simulink model "FPC"  (R2024b)
settings: Solver=FixedStepAuto  StartTime=0.0  StopTime=2.4  FixedStep=1e-5  RelTol=1e-3
values from neighbouring files (symbols this model uses):
  dam = 0.707    [data_foc_fpc_zhang.mat]
  DeltaLUT = [-1.14384315458 -1.14384315458 -1.14384315458 -1.14384315458 -1.14384315458 -1.14384315458 -1.14384315458 -1.14384315458 -1.14384315458 -1.14384315458 -1.14384315458 -1.14384315458 ... (19481 elements, 121x161)]    [deltaLUT_plain_zhang.mat]
  gama = 0.9    [data_foc_fpc_zhang.mat]
  imd = [-200 -190 -180 -170 -160 -150 -140 -130 -120 -110 -100 -90 ... (41 elements, 1x41)]    [data_foc_fpc_zhang.mat]
  imq = [-200 -180 -160 -140 -120 -100 -80 -60 -40 -20 0 20 ... (21 elements, 1x21)]    [data_foc_fpc_zhang.mat]
  L_grid = [0.220516868128 0.222482404345 0.224447940562 0.226413476779 0.228379012997 0.230344549214 0.232310085431 0.234275621648 0.236241157866 0.238206694083 0.2401722303 0.242137766517 ... (121 elements, 1x121)]    [deltaLUT_plain_zhang.mat]
  L_loss = 0.0001    [data_foc_fpc_zhang.mat]
  Lmidd = [0.0012418475022 0.00124844926594 0.00125505102968 0.00126370970426 0.00127249900958 0.00128126693334 0.00129343475618 0.00129881592306 0.00130559003385 0.00130625690774 0.00129596814237 0.00127902455887 ... (861 elements, 41x21)]    [data_foc_fpc_zhang.mat]
  Lmidq = [-8.03588800241e-05 -7.81376313538e-05 -7.59163826835e-05 -6.79567507785e-05 -6.10868587727e-05 -5.46820183962e-05 -4.43623922788e-05 -2.78718084301e-05 -1.24477686412e-05 4.13620151953e-06 2.37103656882e-05 4.4707150748e-05 ... (861 elements, 41x21)]    [data_foc_fpc_zhang.mat]
  Lmiqq = [0.000622544120709 0.000618884908772 0.000615225696834 0.000593520125188 0.000579858645255 0.000568946837315 0.000562248369566 0.000560456845994 0.000560437513873 0.000561933244764 0.00056023385138 0.000557379247045 ... (861 elements, 41x21)]    [data_foc_fpc_zhang.mat]
  phase_number = 3    [data_foc_fpc_zhang.mat]
  pp = 4    [data_foc_fpc_zhang.mat]
  Psid = [-0.0498528002107 -0.0378839484092 -0.0259882808465 -0.013034575748 3.54716858652e-05 0.0129865277943 0.0255980427761 0.0386444323153 0.0516254468728 0.0646548336102 0.0777195684651 0.0905974700702 ... (861 elements, 41x21)]    [data_foc_fpc_zhang.mat]
  Psiq = [-0.428836914229 -0.429385909203 -0.42997932915 -0.43118839194 -0.431809140992 -0.432336580454 -0.433057103512 -0.432963079787 -0.433296951787 -0.433632934983 -0.43343561964 -0.433301309559 ... (861 elements, 41x21)]    [data_foc_fpc_zhang.mat]
  Rs = 0.015    [data_foc_fpc_zhang.mat]
  T_grid = [-218.679204233 -215.967777854 -213.256351475 -210.544925095 -207.833498716 -205.122072337 -202.410645958 -199.699219578 -196.987793199 -194.27636682 -191.56494044 -188.853514061 ... (161 elements, 1x161)]    [deltaLUT_plain_zhang.mat]
  T_ref = 162    [data_foc_fpc_zhang.mat]
  Ts = 1e-05    [data_foc_fpc_zhang.mat]
undefined symbols (not defined in the file or in its folder): DiscIntNeverNeededParam, k_fw, lambdaLUT_801, T_break_801, UNC, V_dc
libraries: simulink x8, mcbcontrolslib x4, spsdq0toabcLib x2, simulink_extras x2, eeTransforms x1, spsabctodq0Lib x1, mcbplantlib x1
settings Model: Creator=zhang5  LastModifiedBy=zhang5
settings DataIOCC: ReturnWorkspaceOutputs=off

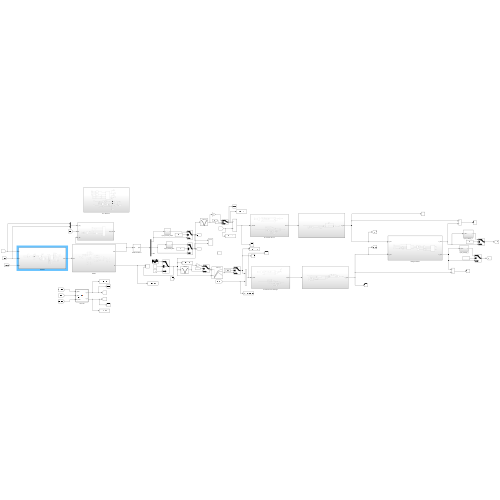
[thumbnail: Simulink's stored preview of the top-level diagram]
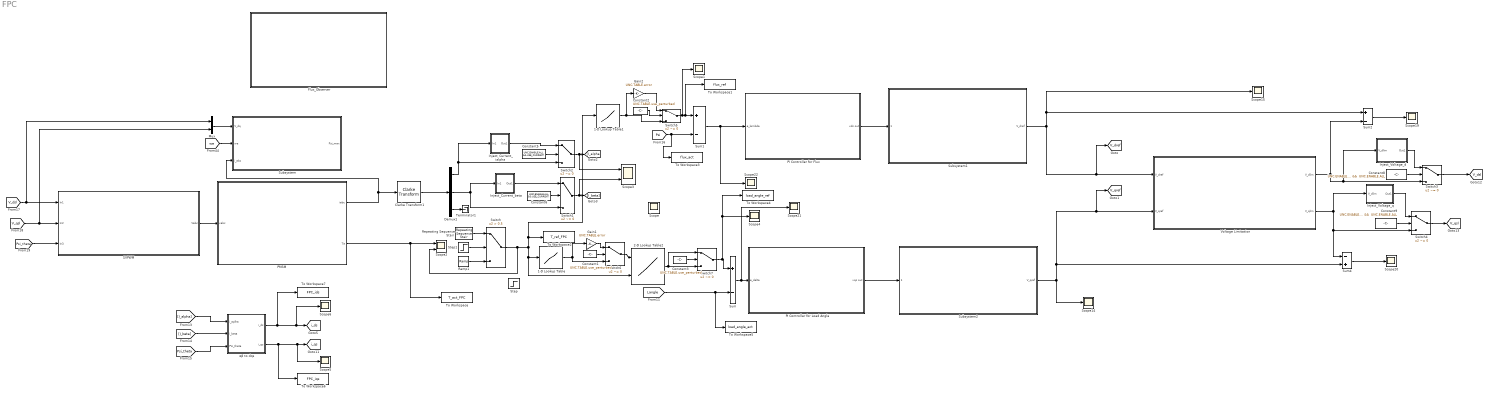
== system FPC ==
  1-D Lookup Table : Lookup_n-D  NumberOfTableDimensions=1  BreakpointsForDimension1=T_break_801  Table=lambdaLUT_801  InternalRulePriority=Speed  RndMeth=Simplest
  1-D Lookup Table1 : Lookup_n-D  NumberOfTableDimensions=1  BreakpointsForDimension1=T_break_801  Table=lambdaLUT_801  InternalRulePriority=Speed  RndMeth=Simplest
  2-D Lookup Table2 : Lookup_n-D  BreakpointsForDimension1=L_grid  BreakpointsForDimension2=T_grid  Table=DeltaLUT  InternalRulePriority=Speed  RndMeth=Simplest
      settings: InputPortMap=u0,u1
  Clarke Transform1 : eeTransforms/Clarke Transform  PowerInvariant=off
      settings: LibrarySourceBlock=|
      | ee_sl_lib/Mathematical
      | Transforms/Clarke Transform
  Constant1 : Constant  Value=UNC.TABLE.use_perturbed
  Constant2 : Constant  Value=UNC.TABLE.use_perturbed
  Constant3 : Constant  Value=UNC.TABLE.use_perturbed
  Constant5 : Constant  Value="UNC.ENABLE.ALL   && USE_CURRENT"
  Constant6 : Constant  Value="UNC.ENABLE.ALL   && USE_CURRENT"
  Constant8 : Constant  Value="UNC.ENABLE.EXEC_DELAY &&  UNC.ENABLE.ALL"
  Constant9 : Constant  Value="UNC.ENABLE.EXEC_DELAY &&  UNC.ENABLE.ALL"
  Demux1 : Demux  Outputs=3
  "Flux_Observer  " : Subsystem
  Gain1 : Gain  Gain=UNC.TABLE.error
  Gain2 : Gain  Gain=UNC.TABLE.error
  Inject_Current_beta : Subsystem
  Inject_Current_ialpha : Subsystem
  Inject_Voltage_d : Subsystem
  Inject_Voltage_q : Subsystem
  Mux : Mux  Inputs=2
  PI Controller for Flux : Subsystem
  "PI Controller for Load Angle " : Subsystem
  PMSM : Subsystem
  Ramp1 : simulink/Sources/Ramp  slope=90  start=0  InitialOutput=0
  Repeating Sequence Stair : simulink/Sources/Repeating Sequence Stair  OutValues=[T_ref -T_ref*0.3 -T_ref*1.8 -T_ref T_ref*1.8 T_ref*0.1].'  tsamp=0.4  OutMin=[]  OutMax=[]  OutDataTypeStr=double  OutputDataTypeScalingMode=double  OutDataType=fixdt(0,8)  ConRadixGroup=Best Precision: Vector-wise  OutScaling=2^-12
  SVPWM : Subsystem
  Scope{,1,4..6,14..15,19..22} (11 alike) : Scope
  Scope2 : Scope  NumInputPorts=2
  Scope3 : Scope  NumInputPorts=2
  Step : Step  Time=0.2  After=162  SampleTime=0
  Step1 : Step  Time=0  SampleTime=0
  Subsystem : Subsystem
  Subsystem1 : Subsystem
  Subsystem2 : Subsystem
  Sum : Sum  Inputs=+-
  Sum1 : Sum  Inputs=+-
  Sum2 : Sum  Inputs=+-
  Sum4 : Sum  Inputs=-+
  Switch : Switch  Criteria=u2 > Threshold  Threshold=0.5  SaturateOnIntegerOverflow=off  InputSameDT=off
  Switch{1..7} (7 alike) : Switch  Criteria=u2 ~= 0  SaturateOnIntegerOverflow=off  InputSameDT=off
  Terminator1 : Terminator
  To Workspace : ToWorkspace  VariableName=T_act_FPC  SaveFormat=Structure With Time  SampleTime=-1
  To Workspace1 : ToWorkspace  VariableName=flux_ref  SaveFormat=Structure With Time  SampleTime=-1
  To Workspace2 : ToWorkspace  VariableName=T_ref_FPC  SaveFormat=Structure With Time  SampleTime=-1
  To Workspace3 : ToWorkspace  VariableName=flux_act  SaveFormat=Structure With Time  SampleTime=-1
  To Workspace4 : ToWorkspace  VariableName=load_angle_ref  SaveFormat=Structure With Time  SampleTime=-1
  To Workspace5 : ToWorkspace  VariableName=load_angle_act  SaveFormat=Structure With Time  SampleTime=-1
  To Workspace6 : ToWorkspace  VariableName=FPC_iqs  SaveFormat=Structure With Time  SampleTime=-1
  To Workspace7 : ToWorkspace  VariableName=FPC_ids  SaveFormat=Structure With Time  SampleTime=-1
  Voltage Limitation : Subsystem
  αβ to dqs : MATLAB Function  TreatAsAtomicUnit=on
  tag scope: V_dref=global, V_dsl=global, V_qref=global, V_qsl=global, i_ds=global, i_qs=global
  wires:
  PMSM/1(iabc) -> Subsystem/3(i_abc), Clarke Transform1/1
  PMSM/2(Te) -> To Workspace/1, Scope2/1
  Clarke Transform1/1 -> Demux1/1
  Demux1/3 -> Terminator1/1
  [Langle] -> To Workspace5/1, Sum/2
  Sum/1 -> Scope21/1, "PI Controller for Load Angle "/1(e_delta)
  [I_alpha] -> αβ to dqs/1(i_aplha)
  [I_beta] -> αβ to dqs/2(i_beta)
  [Psi_theta] -> αβ to dqs/3(Psi_theta)
  αβ to dqs/1(i_ds) -> To Workspace7/1, Scope6/1, [i_ds]
  αβ to dqs/2(i_qs) -> To Workspace6/1, Scope5/1, [i_qs]
  "PI Controller for Load Angle "/1(vqs out) -> Subsystem2/1(" ")
  Subsystem2/1(V_qref) -> [V_qref], Voltage Limitation/2(V_qref), Sum4/2, Scope14/1
  [Psi] -> To Workspace3/1, Sum1/2
  PI Controller for Flux/1(vds out) -> Subsystem1/1(" ")
  Voltage Limitation/1(V_dlim) -> Inject_Voltage_d/1(V_dlim), Switch3/3, Sum2/2
  Sum2/1 -> Scope19/1
  Sum4/1 -> Scope20/1
  Step1/1 -> Switch/2
  Ramp1/1 -> Switch/3
  Repeating Sequence Stair/1 -> Switch/1
  Sum1/1 -> PI Controller for Flux/1(e_lambda), Scope22/1
  Inject_Current_ialpha/1(Out1) -> Switch2/1
  Constant5/1 -> Switch2/2
  Demux1/1 -> Inject_Current_ialpha/1(In1), Switch2/3
  Switch2/1 -> Scope3/1, [I_alpha]
  Demux1/2 -> Switch1/3, Inject_Current_beta/1(In1)
  Constant6/1 -> Switch1/2
  Inject_Current_beta/1(Out1) -> Switch1/1
  Switch1/1 -> Scope3/2, [I_beta]
  Inject_Voltage_d/1(Out1) -> Switch3/1
  Constant8/1 -> Switch3/2
  Switch3/1 -> [V_dsl]
  Constant9/1 -> Switch4/2
  Inject_Voltage_q/1(Out1) -> Switch4/1
  Voltage Limitation/2(V_qlim) -> Switch4/3, Sum4/1, Inject_Voltage_q/1(V_dlim)
  Switch4/1 -> [V_qsl]
  [Psi_theta] -> SVPWM/3(In3)
  [V_dsl] -> Mux/1, SVPWM/1(In1)
  Mux/1 -> Subsystem/1(V_dq)
  [we] -> Subsystem/2(we)
  [V_qsl] -> Mux/2, SVPWM/2(In2)
  SVPWM/1(Vabc) -> PMSM/1(vabc)
  Subsystem1/1(V_dref) -> Sum2/1, Scope15/1, [V_dref], Voltage Limitation/1(V_dref)
  Switch/1 -> Scope2/2, 1-D Lookup Table1/1, To Workspace2/1, 2-D Lookup Table2/2, 1-D Lookup Table/1
  Gain2/1 -> Switch5/1
  Constant2/1 -> Switch5/2
  1-D Lookup Table1/1 -> Gain2/1, Switch5/3
  Switch5/1 -> Scope1/1, To Workspace1/1, Sum1/1
  Switch6/1 -> 2-D Lookup Table2/1
  Constant1/1 -> Switch6/2
  1-D Lookup Table/1 -> Gain1/1, Switch6/3
  Gain1/1 -> Switch6/1
  Switch7/1 -> Scope4/1, To Workspace4/1, Sum/1
  2-D Lookup Table2/1 -> Switch7/1, Switch7/3
  Constant3/1 -> Switch7/2

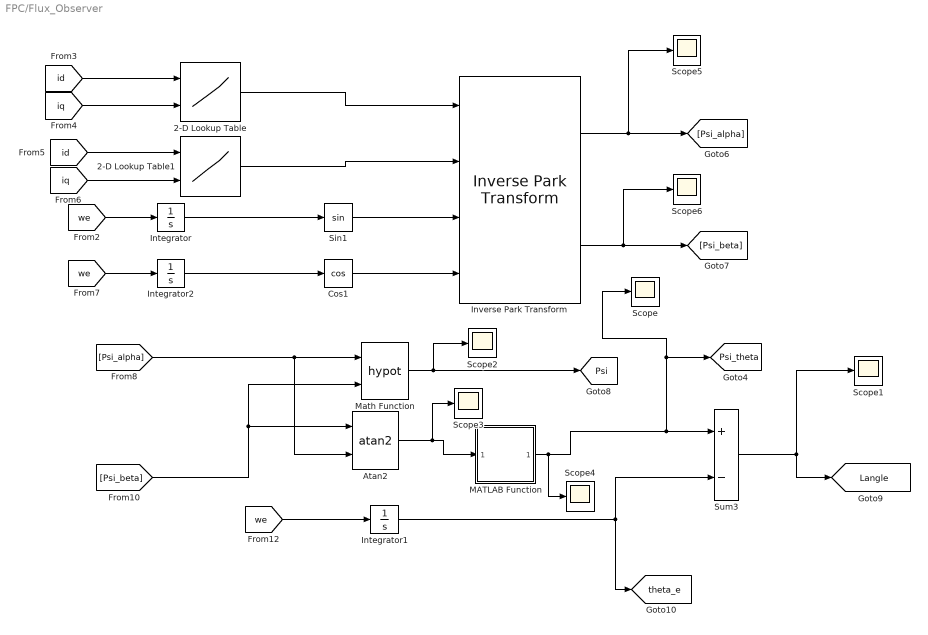
== system FPC/Flux_Observer   ==
  2-D Lookup Table : Lookup_n-D  BreakpointsForDimension1=imd  BreakpointsForDimension2=imq  Table=Psid  InternalRulePriority=Speed  RndMeth=Simplest
      settings: InputPortMap=u0,u1
  2-D Lookup Table1 : Lookup_n-D  BreakpointsForDimension1=imd  BreakpointsForDimension2=imq  Table=Psiq  InternalRulePriority=Speed  RndMeth=Simplest
      settings: InputPortMap=u0,u1
  Atan2 : Trigonometry  Operator=atan2
  Cos1 : Trigonometry  Operator=cos
  Integrator : Integrator
  Integrator1 : Integrator
  Integrator2 : Integrator
  Inverse Park Transform : mcbcontrolslib/Inverse Park Transform  PhaseInput=Two inputs  AxisAlignment=D-axis  ThetaInput=Sine and Cosine electrical position  AngleInput=Per-unit  N_points=1024
      settings: LibrarySourceBlock=mcblib/Controls/Math Transforms/Inverse Park Transform
  MATLAB Function : MATLAB Function  TreatAsAtomicUnit=on
  Math Function : Math  Operator=hypot
  Scope{,1..6} (7 alike) : Scope
  Sin1 : Trigonometry
  Sum3 : Sum  Inputs=+-
  tag scope: Langle=global, Psi=global, Psi_theta=global, theta_e=global
  wires:
  [id] -> 2-D Lookup Table1/1
  MATLAB Function/1(theta_u) -> Scope4/1, [Psi_theta], Scope/1, Sum3/1
  Inverse Park Transform/1 -> Scope5/1, [Psi_alpha]
  [Psi_alpha] -> Atan2/2, Math Function/1
  Integrator2/1 -> Cos1/1
  2-D Lookup Table1/1 -> Inverse Park Transform/2
  [Psi_beta] -> Atan2/1, Math Function/2
  Sin1/1 -> Inverse Park Transform/3
  Integrator/1 -> Sin1/1
  Cos1/1 -> Inverse Park Transform/4
  Integrator1/1 -> [theta_e], Sum3/2
  [we] -> Integrator1/1
  Math Function/1 -> Scope2/1, [Psi]
  Inverse Park Transform/2 -> Scope6/1, [Psi_beta]
  Sum3/1 -> [Langle], Scope1/1
  [iq] -> 2-D Lookup Table/2
  2-D Lookup Table/1 -> Inverse Park Transform/1
  [iq] -> 2-D Lookup Table1/2
  [we] -> Integrator/1
  [we] -> Integrator2/1
  [id] -> 2-D Lookup Table/1
  Atan2/1 -> Scope3/1, MATLAB Function/1(theta_w)

== system FPC/Inject_Current_beta ==
  In1 : Inport
  Band-Limited White Noise : simulink/Sources/Band-Limited White Noise  Cov=UNC.CURR.noise_psd  Ts=1e-5  seed=[23341]
  Bias : Bias  Bias=UNC.CURR.bias_alpha  SaturateOnIntegerOverflow=off
  Quantizer : Quantizer  QuantizationInterval=UNC.CURR.quant
  Sum4 : Sum
  Out1 : Outport
  wires:
  Sum4/1 -> Quantizer/1
  Quantizer/1 -> Out1/1
  In1/1 -> Bias/1
  Bias/1 -> Sum4/1
  Band-Limited White Noise/1 -> Sum4/2

== system FPC/Inject_Current_ialpha ==
  In1 : Inport
  Band-Limited White Noise : simulink/Sources/Band-Limited White Noise  Cov=UNC.CURR.noise_psd  Ts=1e-5  seed=[23341]
  Bias : Bias  Bias=UNC.CURR.bias_alpha  SaturateOnIntegerOverflow=off
  Quantizer : Quantizer  QuantizationInterval=UNC.CURR.quant
  Sum4 : Sum
  Out1 : Outport
  wires:
  Band-Limited White Noise/1 -> Sum4/2
  Bias/1 -> Sum4/1
  In1/1 -> Bias/1
  Quantizer/1 -> Out1/1
  Sum4/1 -> Quantizer/1

== system FPC/Inject_Voltage_d ==
  V_dlim : Inport
  Transport Delay : TransportDelay  DelayTime=UNC.DELAY.ctrl
  Out1 : Outport
  wires:
  Transport Delay/1 -> Out1/1
  V_dlim/1 -> Transport Delay/1

== system FPC/Inject_Voltage_q ==
  V_dlim : Inport
  Transport Delay : TransportDelay  DelayTime=UNC.DELAY.ctrl
  Out1 : Outport
  wires:
  V_dlim/1 -> Transport Delay/1
  Transport Delay/1 -> Out1/1

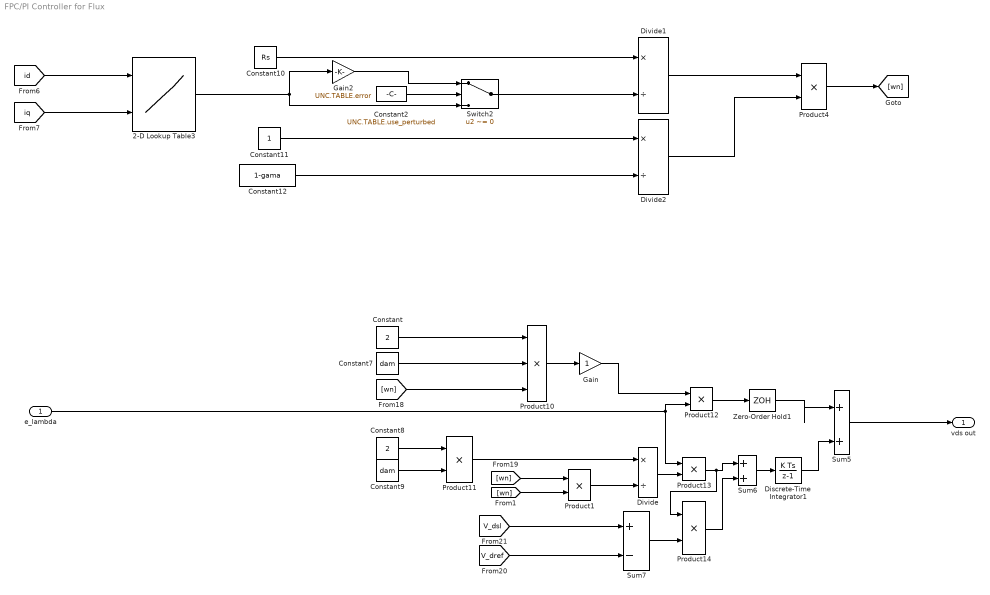
== system FPC/PI Controller for Flux ==
  e_lambda : Inport
  2-D Lookup Table3 : Lookup_n-D  BreakpointsForDimension1=imd  BreakpointsForDimension2=imq  Table=Lmidd  InternalRulePriority=Speed  RndMeth=Simplest
      settings: InputPortMap=u0,u1
  Constant : Constant  Value=2
  Constant10 : Constant  Value=Rs
  Constant11 : Constant
  Constant12 : Constant  Value=1-gama
  Constant2 : Constant  Value=UNC.TABLE.use_perturbed
  Constant7 : Constant  Value=dam
  Constant8 : Constant  Value=2
  Constant9 : Constant  Value=dam
  Discrete-Time Integrator1 : DiscreteIntegrator  SampleTime=Ts  ICPrevOutput=DiscIntNeverNeededParam  ICPrevScaledInput=DiscIntNeverNeededParam
  Divide : Product  Inputs=*/
  Divide1 : Product  Inputs=*/
  Divide2 : Product  Inputs=*/
  Gain : Gain
  Gain2 : Gain  Gain=UNC.TABLE.error
  Product{1,4,11..14} (6 alike) : Product
  Product10 : Product  Inputs=3
  Sum5 : Sum  Inputs=|++
  Sum6 : Sum
  Sum7 : Sum  Inputs=+-
  Switch2 : Switch  Criteria=u2 ~= 0  SaturateOnIntegerOverflow=off  InputSameDT=off
  Zero-Order Hold1 : ZeroOrderHold  SampleTime=Ts
  vds out : Outport
  wires:
  Divide/1 -> Product13/2
  Product12/1 -> Zero-Order Hold1/1
  e_lambda/1 -> Product12/2, Product13/1
  Product10/1 -> Gain/1
  Product11/1 -> Divide/1
  Constant9/1 -> Product11/2
  Constant8/1 -> Product11/1
  [wn] -> Product10/3
  Constant7/1 -> Product10/2
  Constant/1 -> Product10/1
  Sum5/1 -> vds out/1
  Discrete-Time Integrator1/1 -> Sum5/2
  Zero-Order Hold1/1 -> Sum5/1
  Constant12/1 -> Divide2/2
  Divide2/1 -> Product4/2
  Constant11/1 -> Divide2/1
  Divide1/1 -> Product4/1
  [id] -> 2-D Lookup Table3/1
  [iq] -> 2-D Lookup Table3/2
  Constant10/1 -> Divide1/1
  Sum6/1 -> Discrete-Time Integrator1/1
  Product13/1 -> Product14/1, Sum6/1
  Sum7/1 -> Product14/2
  [V_dsl] -> Sum7/1
  [V_dref] -> Sum7/2
  Product14/1 -> Sum6/2
  Product4/1 -> [wn]
  Gain/1 -> Product12/1
  Constant2/1 -> Switch2/2
  Gain2/1 -> Switch2/1
  2-D Lookup Table3/1 -> Switch2/3, Gain2/1
  Switch2/1 -> Divide1/2
  [wn] -> Product1/1
  Product1/1 -> Divide/2
  [wn] -> Product1/2

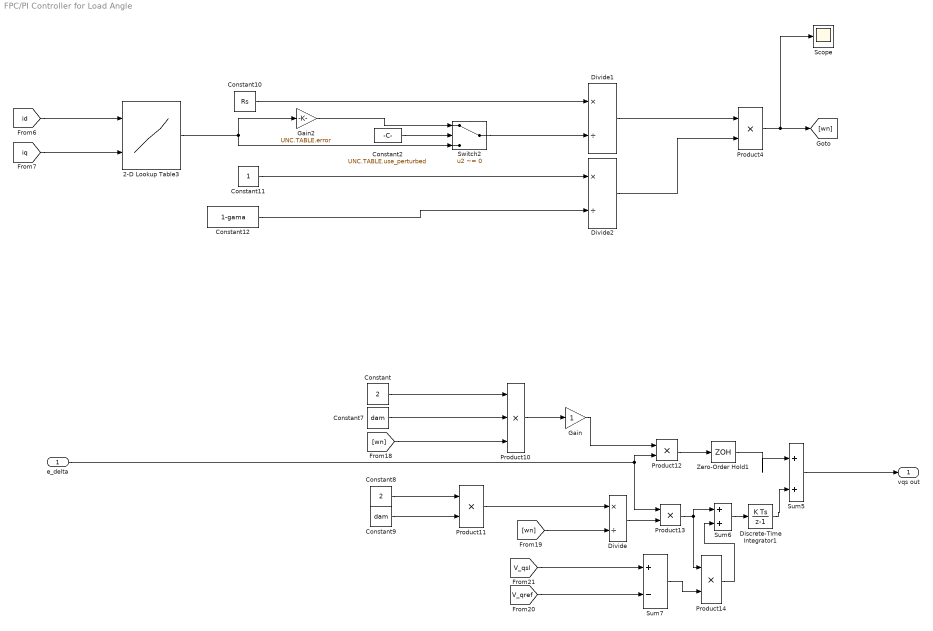
== system FPC/PI Controller for Load Angle  ==
  e_delta : Inport
  2-D Lookup Table3 : Lookup_n-D  BreakpointsForDimension1=imd  BreakpointsForDimension2=imq  Table=Lmiqq  InternalRulePriority=Speed  RndMeth=Simplest
      settings: InputPortMap=u0,u1
  Constant : Constant  Value=2
  Constant10 : Constant  Value=Rs
  Constant11 : Constant
  Constant12 : Constant  Value=1-gama
  Constant2 : Constant  Value=UNC.TABLE.use_perturbed
  Constant7 : Constant  Value=dam
  Constant8 : Constant  Value=2
  Constant9 : Constant  Value=dam
  Discrete-Time Integrator1 : DiscreteIntegrator  SampleTime=Ts  ICPrevOutput=DiscIntNeverNeededParam  ICPrevScaledInput=DiscIntNeverNeededParam
  Divide : Product  Inputs=*/
  Divide1 : Product  Inputs=*/
  Divide2 : Product  Inputs=*/
  Gain : Gain
  Gain2 : Gain  Gain=UNC.TABLE.error
  Product10 : Product  Inputs=3
  Product{4,11..14} (5 alike) : Product
  Scope : Scope
  Sum5 : Sum  Inputs=|++
  Sum6 : Sum
  Sum7 : Sum  Inputs=+-
  Switch2 : Switch  Criteria=u2 ~= 0  SaturateOnIntegerOverflow=off  InputSameDT=off
  Zero-Order Hold1 : ZeroOrderHold  SampleTime=Ts
  vqs out : Outport
  wires:
  Constant10/1 -> Divide1/1
  [iq] -> 2-D Lookup Table3/2
  [id] -> 2-D Lookup Table3/1
  Divide1/1 -> Product4/1
  Product4/1 -> Scope/1, [wn]
  Constant11/1 -> Divide2/1
  Divide2/1 -> Product4/2
  Constant12/1 -> Divide2/2
  Zero-Order Hold1/1 -> Sum5/1
  Discrete-Time Integrator1/1 -> Sum5/2
  Sum5/1 -> vqs out/1
  Constant/1 -> Product10/1
  Constant7/1 -> Product10/2
  [wn] -> Product10/3
  Constant8/1 -> Product11/1
  Constant9/1 -> Product11/2
  Product11/1 -> Divide/1
  [wn] -> Divide/2
  Product10/1 -> Gain/1
  e_delta/1 -> Product13/1, Product12/2
  Product12/1 -> Zero-Order Hold1/1
  Divide/1 -> Product13/2
  Product13/1 -> Product14/1, Sum6/1
  [V_qref] -> Sum7/2
  [V_qsl] -> Sum7/1
  Sum7/1 -> Product14/2
  Sum6/1 -> Discrete-Time Integrator1/1
  Product14/1 -> Sum6/2
  Gain/1 -> Product12/1
  Constant2/1 -> Switch2/2
  Gain2/1 -> Switch2/1
  2-D Lookup Table3/1 -> Switch2/3, Gain2/1
  Switch2/1 -> Divide1/2

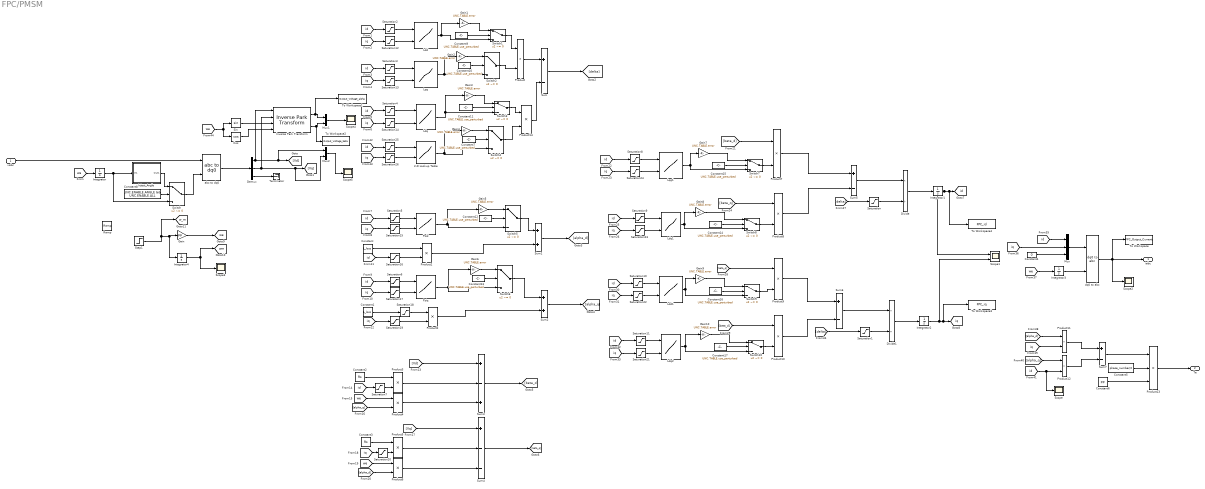
== system FPC/PMSM ==
  vabc : Inport
  2-D Lookup Table : Lookup_n-D  BreakpointsForDimension1=imd  BreakpointsForDimension2=imq  Table=Lmidq  ExtrapMethod=Clip  UseLastTableValue=on  InternalRulePriority=Speed  RndMeth=Simplest
      settings: InputPortMap=u0,u1
  Constant : Constant  Value=L_loss
  Constant1 : Constant  Value=L_loss
  Constant{7,9..17} (10 alike) : Constant  Value=UNC.TABLE.use_perturbed
  Constant2 : Constant  Value=Rs
  Constant3 : Constant  Value=Rs
  Constant4 : Constant  Value=0
  Constant5 : Constant  Value=phase_number/2
  Constant6 : Constant  Value=pp
  Constant8 : Constant  Value=UNC.ENABLE.ANGLE && UNC.ENABLE.ALL
  Cos : Trigonometry  Operator=cos
  Demux : Demux  Outputs=3
  Divide : Product  Inputs=*/
  Divide1 : Product  Inputs=*/
  Gain : Gain  Gain=pp
  Gain{1..10} (10 alike) : Gain  Gain=UNC.TABLE.error
  Inject_Angle : Subsystem
  Integrator : Integrator  UpperSaturationLimit=pi  LowerSaturationLimit=-pi
  Integrator1 : Integrator
  Integrator2 : Integrator
  Integrator3 : Integrator  UpperSaturationLimit=pi  LowerSaturationLimit=-pi
  Integrator4 : Integrator
  Inverse Park Transform : mcbcontrolslib/Inverse Park Transform  PhaseInput=Two inputs  AxisAlignment=D-axis  ThetaInput=Sine and Cosine electrical position  AngleInput=Per-unit  N_points=1024
      settings: LibrarySourceBlock=mcbhdllib/Controls/Math Transforms/Inverse Park Transform
  Ldd : Lookup_n-D  BreakpointsForDimension1=imd  BreakpointsForDimension2=imq  Table=Lmidd  ExtrapMethod=Clip  UseLastTableValue=on  InternalRulePriority=Speed  RndMeth=Simplest
      settings: InputPortMap=u0,u1
  Ldd1 : Lookup_n-D  BreakpointsForDimension1=imd  BreakpointsForDimension2=imq  Table=Lmidd  ExtrapMethod=Clip  UseLastTableValue=on  InternalRulePriority=Speed  RndMeth=Simplest
      settings: InputPortMap=u0,u1
  Ldq : Lookup_n-D  BreakpointsForDimension1=imd  BreakpointsForDimension2=imq  Table=Lmidq  ExtrapMethod=Clip  UseLastTableValue=on  InternalRulePriority=Speed  RndMeth=Simplest
      settings: InputPortMap=u0,u1
  Ldq1 : Lookup_n-D  BreakpointsForDimension1=imd  BreakpointsForDimension2=imq  Table=Lmidq  ExtrapMethod=Clip  UseLastTableValue=on  InternalRulePriority=Speed  RndMeth=Simplest
      settings: InputPortMap=u0,u1
  Ldq2 : Lookup_n-D  BreakpointsForDimension1=imd  BreakpointsForDimension2=imq  Table=Lmidq  ExtrapMethod=Clip  UseLastTableValue=on  InternalRulePriority=Speed  RndMeth=Simplest
      settings: InputPortMap=u0,u1
  Lqq : Lookup_n-D  BreakpointsForDimension1=imd  BreakpointsForDimension2=imq  Table=Lmiqq  ExtrapMethod=Clip  UseLastTableValue=on  InternalRulePriority=Speed  RndMeth=Simplest
      settings: InputPortMap=u0,u1
  Lqq1 : Lookup_n-D  BreakpointsForDimension1=imd  BreakpointsForDimension2=imq  Table=Lmiqq  ExtrapMethod=Clip  UseLastTableValue=on  InternalRulePriority=Speed  RndMeth=Simplest
      settings: InputPortMap=u0,u1
  Mux : Mux  Inputs=3
  Mux1 : Mux  Inputs=2
  Mux2 : Mux  Inputs=2
  Product{,1..12,14} (14 alike) : Product
  Product13 : Product  Inputs=3
  Psid : Lookup_n-D  BreakpointsForDimension1=imd  BreakpointsForDimension2=imq  Table=Psid  ExtrapMethod=Clip  UseLastTableValue=on  InternalRulePriority=Speed  RndMeth=Simplest
      settings: InputPortMap=u0,u1
  Psiq : Lookup_n-D  BreakpointsForDimension1=imd  BreakpointsForDimension2=imq  Table=Psiq  ExtrapMethod=Clip  UseLastTableValue=on  InternalRulePriority=Speed  RndMeth=Simplest
      settings: InputPortMap=u0,u1
  Ramp : simulink/Sources/Ramp  slope=8.9757  start=0  InitialOutput=0
  Saturation : Saturate  UpperLimit=10000000000000000000000  LowerLimit=1e-6
  Saturation1 : Saturate  UpperLimit=10000000000000000000000  LowerLimit=1e-6
  Saturation{2..11,13..26} (24 alike) : Saturate  UpperLimit=200  LowerLimit=-200
  Saturation12 : Saturate
  Scope{,2..5} (5 alike) : Scope
  Scope1 : Scope  NumInputPorts=2
  Sin : Trigonometry
  Step1 : Step  Time=5  Before=10.4720 * 2  After=10.4720*1.2  SampleTime=0
  Sum{,5..7} (4 alike) : Sum  Inputs=+-
  Sum1 : Sum
  Sum2 : Sum
  Sum3 : Sum  Inputs=+-+
  Sum4 : Sum  Inputs=+--
  Switch{,1..10} (11 alike) : Switch  Criteria=u2 ~= 0  SaturateOnIntegerOverflow=off  InputSameDT=off
  Terminator : Terminator
  To Workspace : ToWorkspace  VariableName=FPC_Output_Current  SaveFormat=Timeseries  SampleTime=-1
  To Workspace1 : ToWorkspace  VariableName=Output_Voltage_alpha  SaveFormat=Structure With Time  SampleTime=-1
  To Workspace2 : ToWorkspace  VariableName=Output_Voltage_beta  SaveFormat=Structure With Time  SampleTime=-1
  To Workspace3 : ToWorkspace  VariableName=FPC_iq  SaveFormat=Structure With Time  SampleTime=-1
  To Workspace4 : ToWorkspace  VariableName=FPC_id  SaveFormat=Structure With Time  SampleTime=-1
  abc to dq0 : spsabctodq0Lib/abc to dq0  Alignment=Aligned with phase A axis
  dq0 to abc : spsdq0toabcLib/dq0 to abc  Alignment=Aligned with phase A axis
  iabc : Outport
  Te : Outport  Port=2
  tag scope: id=global, iq=global, w_m=global, we=global, wm=global
  wires:
  Product1/1 -> Sum1/2
  abc to dq0/1 -> Demux/1
  Demux/2 -> Inverse Park Transform/2, Mux2/2, [Vq]
  Demux/1 -> Inverse Park Transform/1, Mux2/1, [Vd]
  Product2/1 -> Sum2/2
  Saturation26/1 -> 2-D Lookup Table/2
  Saturation25/1 -> 2-D Lookup Table/1
  [iq] -> Saturation26/1
  [id] -> Saturation25/1
  Saturation24/1 -> Lqq1/2
  Saturation23/1 -> Ldq1/2
  Saturation22/1 -> Ldd1/2
  Saturation21/1 -> Ldq2/2
  Saturation20/1 -> Product5/2
  Saturation19/1 -> Product2/2
  Saturation18/1 -> Product2/1
  Saturation17/1 -> Psiq/2
  Saturation16/1 -> Product1/2
  Saturation15/1 -> Psid/2
  Saturation14/1 -> Ldq/2
  Saturation13/1 -> Lqq/2
  Saturation12/1 -> Ldd/2
  Saturation11/1 -> Ldq2/1
  Saturation10/1 -> Ldd1/1
  Saturation9/1 -> Ldq1/1
  Saturation8/1 -> Lqq1/1
  Saturation7/1 -> Product3/2
  Saturation6/1 -> Psiq/1
  Saturation5/1 -> Psid/1
  Saturation4/1 -> Ldq/1
  Saturation3/1 -> Lqq/1
  Saturation2/1 -> Ldd/1
  Saturation1/1 -> Divide1/2
  Saturation/1 -> Divide/2
  Product13/1 -> Te/1
  Constant6/1 -> Product13/3
  Constant5/1 -> Product13/2
  Sum7/1 -> Product13/1
  Product12/1 -> Sum7/2
  [id] -> Product12/2, Scope/1
  [alpha_q] -> Product12/1
  Product11/1 -> Sum7/1
  [iq] -> Product11/2
  [alpha_d] -> Product11/1
  [beta_q] -> Product9/1
  [iq] -> Saturation22/1
  Sum/1 -> [delta]
  Constant/1 -> Product1/1
  Integrator1/1 -> Scope1/1, To Workspace4/1, [id]
  [delta] -> Saturation1/1
  [Vd] -> Sum3/1
  [id] -> Saturation5/1
  [id] -> Saturation11/1
  Sum1/1 -> [alpha_d]
  Sum4/1 -> [beta_q]
  [alpha_q] -> Product4/2
  Sum3/1 -> [beta_d]
  [we] -> Product6/1
  Sum6/1 -> Divide1/1
  Product/1 -> Sum/1
  [iq] -> Saturation23/1
  [we] -> Product4/1
  [id] -> Mux/1
  Product10/1 -> Sum6/2
  Constant1/1 -> Saturation18/1
  Product5/1 -> Sum4/2
  Product9/1 -> Sum6/1
  Divide/1 -> Integrator1/1
  [iq] -> Mux/2
  [id] -> Saturation8/1
  [beta_d] -> Product7/1
  Integrator2/1 -> To Workspace3/1, [iq], Scope1/2
  Integrator3/1 -> dq0 to abc/2
  [beta_q] -> Product8/1
  Gain/1 -> [we]
  Product3/1 -> Sum3/2
  Product8/1 -> Sum5/2
  Sum5/1 -> Divide/1
  [id] -> Saturation7/1
  [delta] -> Saturation/1
  [we] -> Integrator3/1
  [iq] -> Saturation20/1
  [id] -> Saturation4/1
  Product14/1 -> Sum/2
  Sum2/1 -> [alpha_q]
  Product7/1 -> Sum5/1
  [iq] -> Saturation24/1
  [id] -> Saturation3/1
  [iq] -> Saturation13/1
  Product6/1 -> Sum4/3
  [id] -> Saturation9/1
  Mux/1 -> dq0 to abc/1
  [iq] -> Saturation14/1
  [alpha_d] -> Product6/2
  Divide1/1 -> Integrator2/1
  [Vq] -> Sum4/1
  [id] -> Saturation6/1
  Constant4/1 -> Mux/3
  dq0 to abc/1 -> To Workspace/1, iabc/1, Scope2/1
  Demux/3 -> Terminator/1
  [id] -> Saturation10/1
  [we] -> Integrator/1
  [beta_d] -> Product10/1
  [id] -> Saturation2/1
  Constant3/1 -> Product5/1
  [id] -> Saturation16/1
  [iq] -> Saturation15/1
  [iq] -> Saturation19/1
  Product4/1 -> Sum3/3
  Constant2/1 -> Product3/1
  [iq] -> Saturation21/1
  [iq] -> Saturation12/1
  [iq] -> Saturation17/1
  vabc/1 -> abc to dq0/1
  Step1/1 -> Gain/1, Integrator4/1, [w_m]
  Constant8/1 -> Switch/2
  Inject_Angle/1(Out1) -> Switch/1
  Integrator/1 -> Switch/3, Inject_Angle/1(In1)
  Integrator4/1 -> Scope3/1, [wm]
  Switch/1 -> abc to dq0/2
  Constant10/1 -> Switch2/2
  Switch2/1 -> Product/2
  Gain2/1 -> Switch2/1
  Gain1/1 -> Switch1/1
  Constant9/1 -> Switch1/2
  Ldd/1 -> Gain1/1, Switch1/3
  Lqq/1 -> Switch2/3, Gain2/1
  Switch1/1 -> Product/1
  2-D Lookup Table/1 -> Gain4/1, Switch4/3
  Ldq/1 -> Switch3/3, Gain3/1
  Constant11/1 -> Switch3/2
  Gain3/1 -> Switch3/1
  Gain4/1 -> Switch4/1
  Switch4/1 -> Product14/2
  Constant7/1 -> Switch4/2
  Switch3/1 -> Product14/1
  Constant12/1 -> Switch5/2
  Gain5/1 -> Switch5/1
  Psid/1 -> Gain5/1, Switch5/3
  Switch5/1 -> Sum1/1
  Switch6/1 -> Sum2/1
  Psiq/1 -> Switch6/3, Gain6/1
  Gain6/1 -> Switch6/1
  Constant13/1 -> Switch6/2
  Constant15/1 -> Switch7/2
  Gain7/1 -> Switch7/1
  Lqq1/1 -> Switch7/3, Gain7/1
  Switch7/1 -> Product7/2
  Ldq1/1 -> Gain8/1, Switch8/3
  Gain8/1 -> Switch8/1
  Constant14/1 -> Switch8/2
  Switch8/1 -> Product8/2
  Constant16/1 -> Switch9/2
  Gain9/1 -> Switch9/1
  Ldd1/1 -> Switch9/3, Gain9/1
  Switch9/1 -> Product9/2
  Ldq2/1 -> Switch10/3, Gain10/1
  Gain10/1 -> Switch10/1
  Constant17/1 -> Switch10/2
  Switch10/1 -> Product10/2
  Sin/1 -> Inverse Park Transform/3
  [we] -> Cos/1, Sin/1
  Cos/1 -> Inverse Park Transform/4
  Inverse Park Transform/1 -> To Workspace1/1, Mux1/1
  Inverse Park Transform/2 -> To Workspace2/1, Mux1/2
  Mux1/1 -> Scope4/1
  Mux2/1 -> Scope5/1

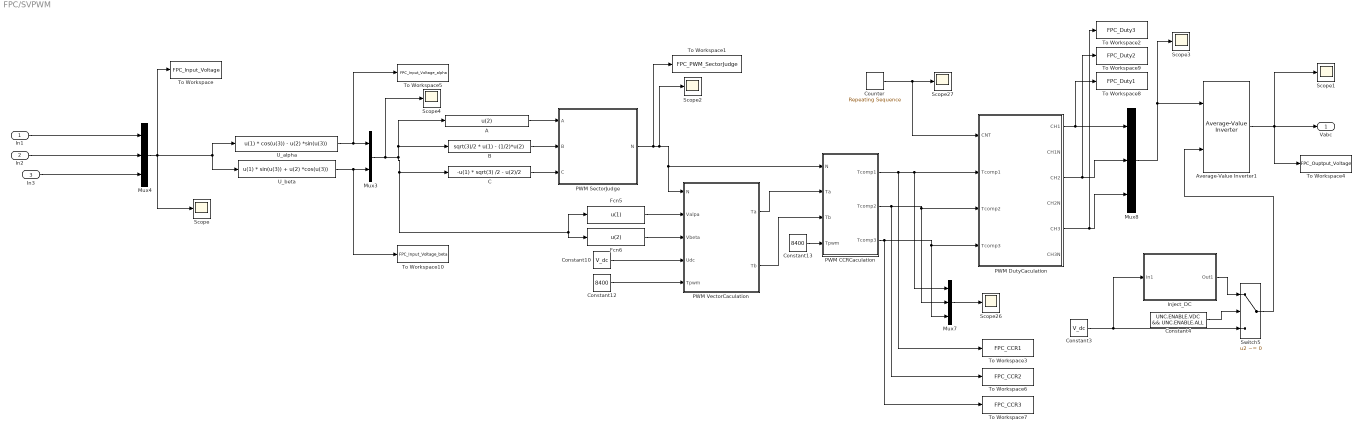
== system FPC/SVPWM ==
  In1 : Inport
  In2 : Inport  Port=2
  In3 : Inport  Port=3
  A : Fcn  Expr=u(2)
  Average-Value Inverter1 : mcbplantlib/Average-Value Inverter
      settings: LibrarySourceBlock=mcblib/Electrical Systems/Inverters/Average-Value Inverter
  B : Fcn  Expr=sqrt(3)/2 * u(1) - (1/2)*u(2)
  C : Fcn  Expr=-u(1) * sqrt(3) /2 - u(2)/2
  Constant10 : Constant  Value=V_dc
  Constant12 : Constant  Value=8400
  Constant13 : Constant  Value=8400
  Constant3 : Constant  Value=V_dc
  Constant4 : Constant  Value=UNC.ENABLE.VDC && UNC.ENABLE.ALL
  Counter : simulink/Sources/Repeating Sequence  rep_seq_t=[0 0.00025 0.0005]  rep_seq_y=[0 4200 0]
  Fcn5 : Fcn  Expr=u(1)
  Fcn6 : Fcn  Expr=u(2)
  Inject_DC : Subsystem
  Mux3 : Mux  Inputs=2
  Mux4 : Mux  Inputs=3
  Mux7 : Mux  Inputs=3
  Mux8 : Mux  Inputs=3
  PWM CCRCaculation : MATLAB Function  TreatAsAtomicUnit=on
  PWM DutyCaculation : MATLAB Function  TreatAsAtomicUnit=on
  PWM SectorJudge : MATLAB Function  TreatAsAtomicUnit=on
  PWM VectorCaculation : MATLAB Function  TreatAsAtomicUnit=on
  Scope{,1..4,26..27} (7 alike) : Scope
  Switch5 : Switch  Criteria=u2 ~= 0  SaturateOnIntegerOverflow=off  InputSameDT=off
  To Workspace : ToWorkspace  VariableName=FPC_Input_Voltage  SaveFormat=Structure With Time  SampleTime=-1
  To Workspace1 : ToWorkspace  VariableName=FPC_PWM_SectorJudge  SaveFormat=Structure With Time  SampleTime=-1
  To Workspace10 : ToWorkspace  VariableName=FPC_Input_Voltage_beta  SaveFormat=Structure With Time  SampleTime=-1
  To Workspace2 : ToWorkspace  VariableName=FPC_Duty3  SaveFormat=Structure With Time  SampleTime=-1
  To Workspace3 : ToWorkspace  VariableName=FPC_CCR1  SaveFormat=Structure With Time  SampleTime=-1
  To Workspace4 : ToWorkspace  VariableName=FPC_Ouptput_Voltage  SaveFormat=Structure With Time  SampleTime=-1
  To Workspace5 : ToWorkspace  VariableName=FPC_Input_Voltage_alpha  SaveFormat=Structure With Time  SampleTime=-1
  To Workspace6 : ToWorkspace  VariableName=FPC_CCR2  SaveFormat=Structure With Time  SampleTime=-1
  To Workspace7 : ToWorkspace  VariableName=FPC_CCR3  SaveFormat=Structure With Time  SampleTime=-1
  To Workspace8 : ToWorkspace  VariableName=FPC_Duty1  SaveFormat=Structure With Time  SampleTime=-1
  To Workspace9 : ToWorkspace  VariableName=FPC_Duty2  SaveFormat=Structure With Time  SampleTime=-1
  U_alpha : Fcn  Expr=u(1) * cos(u(3)) - u(2) *sin(u(3))
  U_beta : Fcn  Expr=u(1) * sin(u(3)) + u(2) *cos(u(3))
  Vabc : Outport
  wires:
  PWM CCRCaculation/1(Tcomp1) -> To Workspace3/1, Mux7/1, PWM DutyCaculation/2(Tcomp1)
  PWM DutyCaculation/5(CH3) -> To Workspace2/1, Mux8/3
  Mux3/1 -> Scope4/1, Fcn6/1, Fcn5/1, C/1, A/1, B/1
  B/1 -> PWM SectorJudge/2(B)
  PWM SectorJudge/1(N) -> To Workspace1/1, Scope2/1, PWM VectorCaculation/1(N), PWM CCRCaculation/1(N)
  Mux4/1 -> Scope/1, To Workspace/1, U_beta/1, U_alpha/1
  Constant3/1 -> Switch5/3, Inject_DC/1(In1)
  Counter/1 -> Scope27/1, PWM DutyCaculation/1(CNT)
  Constant4/1 -> Switch5/2
  Inject_DC/1(Out1) -> Switch5/1
  PWM DutyCaculation/1(CH1) -> To Workspace8/1, Mux8/1
  Constant10/1 -> PWM VectorCaculation/4(Udc)
  PWM DutyCaculation/3(CH2) -> To Workspace9/1, Mux8/2
  U_beta/1 -> To Workspace10/1, Mux3/2
  Constant13/1 -> PWM CCRCaculation/4(Tpwm)
  Fcn6/1 -> PWM VectorCaculation/3(Vbeta)
  C/1 -> PWM SectorJudge/3(C)
  A/1 -> PWM SectorJudge/1(A)
  PWM CCRCaculation/2(Tcomp2) -> To Workspace6/1, Mux7/2, PWM DutyCaculation/3(Tcomp2)
  Mux7/1 -> Scope26/1
  U_alpha/1 -> To Workspace5/1, Mux3/1
  Constant12/1 -> PWM VectorCaculation/5(Tpwm)
  PWM VectorCaculation/2(Tb) -> PWM CCRCaculation/3(Tb)
  PWM CCRCaculation/3(Tcomp3) -> To Workspace7/1, Mux7/3, PWM DutyCaculation/4(Tcomp3)
  In1/1 -> Mux4/1
  Switch5/1 -> Average-Value Inverter1/2
  Fcn5/1 -> PWM VectorCaculation/2(Valpa)
  Mux8/1 -> Scope3/1, Average-Value Inverter1/1
  PWM VectorCaculation/1(Ta) -> PWM CCRCaculation/2(Ta)
  In3/1 -> Mux4/3
  In2/1 -> Mux4/2
  Average-Value Inverter1/1 -> Scope1/1, Vabc/1, To Workspace4/1

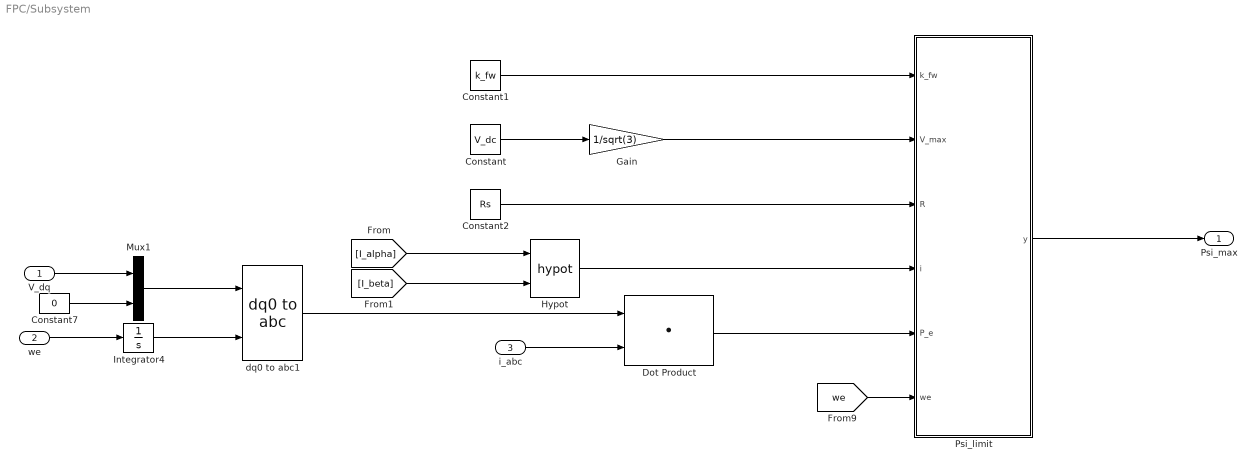
== system FPC/Subsystem ==
  V_dq : Inport
  we : Inport  Port=2
  i_abc : Inport  Port=3
  Constant : Constant  Value=V_dc
  Constant1 : Constant  Value=k_fw
  Constant2 : Constant  Value=Rs
  Constant7 : Constant  Value=0
  Dot Product : DotProduct  OutDataTypeStr=Inherit: Inherit via internal rule
  Gain : Gain  Gain=1/sqrt(3)
  Hypot : Math  Operator=hypot
  Integrator4 : Integrator  UpperSaturationLimit=pi  LowerSaturationLimit=-pi
  Mux1 : Mux  Inputs=2
  Psi_limit : MATLAB Function  TreatAsAtomicUnit=on
  dq0 to abc1 : spsdq0toabcLib/dq0 to abc  Alignment=Aligned with phase A axis
  Psi_max : Outport
  wires:
  Integrator4/1 -> dq0 to abc1/2
  [I_beta] -> Hypot/2
  Dot Product/1 -> Psi_limit/5(P_e)
  Hypot/1 -> Psi_limit/4(i)
  Constant1/1 -> Psi_limit/1(k_fw)
  Mux1/1 -> dq0 to abc1/1
  Psi_limit/1(y) -> Psi_max/1
  Constant7/1 -> Mux1/2
  Constant/1 -> Gain/1
  [we] -> Psi_limit/6(we)
  i_abc/1 -> Dot Product/2
  [I_alpha] -> Hypot/1
  Gain/1 -> Psi_limit/2(V_max)
  dq0 to abc1/1 -> Dot Product/1
  Constant2/1 -> Psi_limit/3(R)
  we/1 -> Integrator4/1
  V_dq/1 -> Mux1/1

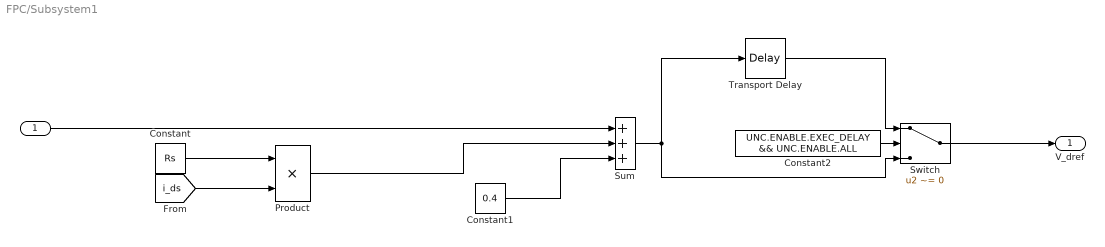
== system FPC/Subsystem1 ==
  " " : Inport
  Constant : Constant  Value=Rs
  Constant1 : Constant  Value=0.4
  Constant2 : Constant  Value=UNC.ENABLE.EXEC_DELAY && UNC.ENABLE.ALL
  Product : Product
  Sum : Sum  Inputs=+++
  Switch : Switch  Criteria=u2 ~= 0  SaturateOnIntegerOverflow=off  InputSameDT=off
  Transport Delay : TransportDelay  DelayTime=UNC.DELAY.ff
  V_dref : Outport
  wires:
  Product/1 -> Sum/2
  Constant/1 -> Product/1
  [i_ds] -> Product/2
  " "/1 -> Sum/1
  Constant1/1 -> Sum/3
  Transport Delay/1 -> Switch/1
  Switch/1 -> V_dref/1
  Sum/1 -> Switch/3, Transport Delay/1
  Constant2/1 -> Switch/2

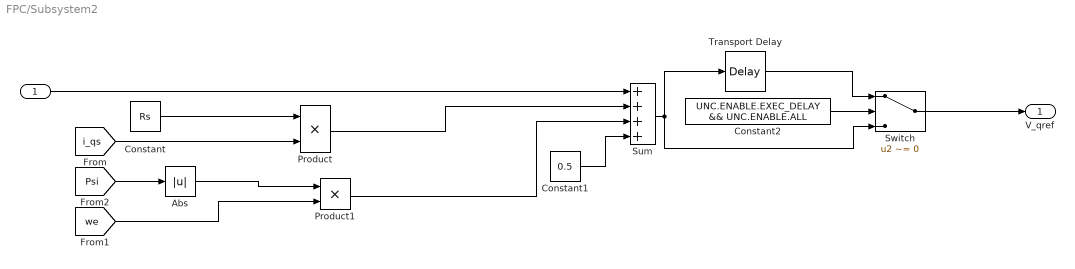
== system FPC/Subsystem2 ==
  " " : Inport
  Abs : Abs  SaturateOnIntegerOverflow=off
  Constant : Constant  Value=Rs
  Constant1 : Constant  Value=0.5
  Constant2 : Constant  Value=UNC.ENABLE.EXEC_DELAY && UNC.ENABLE.ALL
  Product : Product
  Product1 : Product
  Sum : Sum  Inputs=++++
  Switch : Switch  Criteria=u2 ~= 0  SaturateOnIntegerOverflow=off  InputSameDT=off
  Transport Delay : TransportDelay  DelayTime=UNC.DELAY.ff
  V_qref : Outport
  wires:
  Constant/1 -> Product/1
  [i_qs] -> Product/2
  Product/1 -> Sum/2
  Product1/1 -> Sum/3
  [we] -> Product1/2
  [Psi] -> Abs/1
  Abs/1 -> Product1/1
  " "/1 -> Sum/1
  Constant1/1 -> Sum/4
  Constant2/1 -> Switch/2
  Transport Delay/1 -> Switch/1
  Switch/1 -> V_qref/1
  Sum/1 -> Switch/3, Transport Delay/1

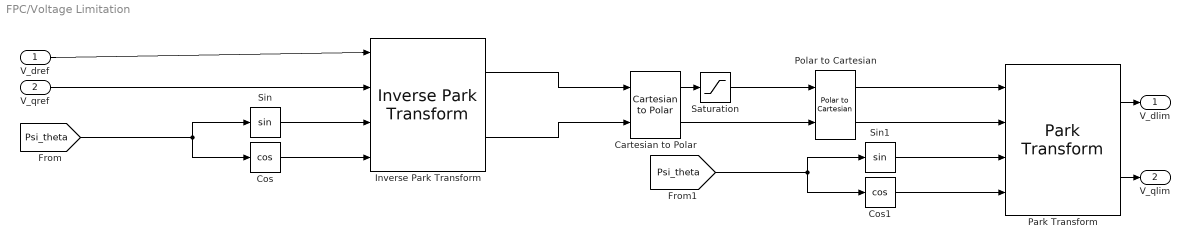
== system FPC/Voltage Limitation ==
  V_dref : Inport
  V_qref : Inport  Port=2
  Cartesian to Polar : simulink_extras/Transformations/Cartesian to Polar
  Cos : Trigonometry  Operator=cos
  Cos1 : Trigonometry  Operator=cos
  Inverse Park Transform : mcbcontrolslib/Inverse Park Transform  PhaseInput=Two inputs  AxisAlignment=D-axis  ThetaInput=Sine and Cosine electrical position  AngleInput=Per-unit  N_points=1024
      settings: LibrarySourceBlock=mcblib/Controls/Math Transforms/Inverse Park Transform
  Park Transform : mcbcontrolslib/Park Transform  PhaseInput=Two inputs  AxisAlignment=D-axis  ThetaInput=Sine and Cosine electrical position  AngleInput=Per-unit  N_points=1024
      settings: LibrarySourceBlock=mcblib/Controls/Math Transforms/Park Transform
  Polar to Cartesian : simulink_extras/Transformations/Polar to Cartesian
  Saturation : Saturate  UpperLimit=V_dc  LowerLimit=0
  Sin : Trigonometry
  Sin1 : Trigonometry
  V_dlim : Outport
  V_qlim : Outport  Port=2
  wires:
  Park Transform/1 -> V_dlim/1
  Cos/1 -> Inverse Park Transform/4
  Cartesian to Polar/2 -> Polar to Cartesian/2
  Polar to Cartesian/2 -> Park Transform/2
  Polar to Cartesian/1 -> Park Transform/1
  Saturation/1 -> Polar to Cartesian/1
  Inverse Park Transform/1 -> Cartesian to Polar/1
  Sin/1 -> Inverse Park Transform/3
  Inverse Park Transform/2 -> Cartesian to Polar/2
  Park Transform/2 -> V_qlim/1
  Cos1/1 -> Park Transform/4
  Cartesian to Polar/1 -> Saturation/1
  V_qref/1 -> Inverse Park Transform/2
  Sin1/1 -> Park Transform/3
  V_dref/1 -> Inverse Park Transform/1
  [Psi_theta] -> Cos1/1, Sin1/1
  [Psi_theta] -> Sin/1, Cos/1

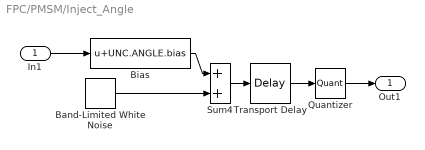
== system FPC/PMSM/Inject_Angle ==
  In1 : Inport
  Band-Limited White Noise : simulink/Sources/Band-Limited White Noise  Cov=UNC.ANGLE.noise  Ts=1e-5  seed=[23341]
  Bias : Bias  Bias=UNC.ANGLE.bias  SaturateOnIntegerOverflow=off
  Quantizer : Quantizer  QuantizationInterval=UNC.ANGLE.quant
  Sum4 : Sum
  Transport Delay : TransportDelay  DelayTime=UNC.ANGLE.delay
  Out1 : Outport
  wires:
  Transport Delay/1 -> Quantizer/1
  Sum4/1 -> Transport Delay/1
  Quantizer/1 -> Out1/1
  In1/1 -> Bias/1
  Bias/1 -> Sum4/1
  Band-Limited White Noise/1 -> Sum4/2

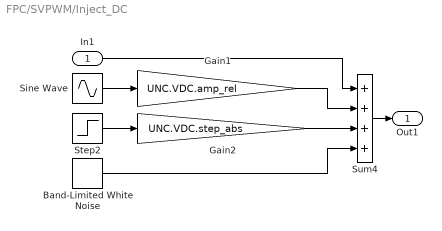
== system FPC/SVPWM/Inject_DC ==
  In1 : Inport
  Band-Limited White Noise : simulink/Sources/Band-Limited White Noise  Cov=UNC.VDC.noise  Ts=1e-5  seed=[23341]
  Gain1 : Gain  Gain=UNC.VDC.amp_rel
  Gain2 : Gain  Gain=UNC.VDC.step_abs
  Sine Wave : Sin  Frequency=2*pi*120  SampleTime=0
  Step2 : Step  Time=0.05  SampleTime=0
  Sum4 : Sum  Inputs=++++
  Out1 : Outport
  wires:
  In1/1 -> Sum4/1
  Gain2/1 -> Sum4/3
  Sine Wave/1 -> Gain1/1
  Step2/1 -> Gain2/1
  Gain1/1 -> Sum4/2
  Band-Limited White Noise/1 -> Sum4/4
  Sum4/1 -> Out1/1

== matlab function FPC/Flux_Observer  /MATLAB Function ==
  settings: updateMethod=DISCRETE
  data: theta_w input; theta_u output
function theta_u = unwrap_angle(theta_w)

persistent last off
if isempty(last); last = theta_w; off = 0; end
d = theta_w - last;
if d >  pi
    off = off - 2*pi;
elseif d < -pi
    off = off + 2*pi;
end
last = theta_w;
theta_u = theta_w + off;   % 这就是“连续角度”
end

== matlab function FPC/Subsystem/Psi_limit ==
  data: k_fw input; y output; V_max input; R input; i input; P_e input; we input
function y = fcn(k_fw, V_max, R, i, P_e, we)

y = k_fw * sqrt(V_max^2 + (R*i)^2 - (4/3)*R*P_e)/we;
end

== matlab function FPC/αβ to dqs ==
  data: i_aplha input; i_ds output; i_beta input; i_qs output; Psi_theta input
function [i_ds, i_qs] = dqs_tranform(i_aplha,i_beta, Psi_theta)

i_ds = cos(Psi_theta) * i_aplha + sin(Psi_theta) * i_beta;
i_qs = -sin(Psi_theta) * i_aplha + cos(Psi_theta) * i_beta;

== matlab function FPC/SVPWM/PWM CCRCaculation ==
  data: N input; Tcomp1 output; Ta input; Tb input; Tpwm input; Tcomp2 output; Tcomp3 output
function [Tcomp1, Tcomp2, Tcomp3] = CCRCaculation(N, Ta, Tb, Tpwm)

Tcomp1 = double(0);
Tcomp2 = double(0);
Tcomp3 = double(0);

Ttemp = Ta + Tb;
if (Ttemp > Tpwm)
    Ta = Ta / Ttemp * Tpwm;
    Tb = Tb / Ttemp * Tpwm;
end
value1 = (Tpwm - Ta - Tb) / 4.0;
value2 = value1 + Ta / 2.0;
value3 = value2 + Tb / 2.0;

switch(N)
    case 3
        Tcomp1 = value1;
        Tcomp2 = value2;
        Tcomp3 = value3;
    case 1
        Tcomp1 = value2;
        Tcomp2 = value1;
        Tcomp3 = value3;

    case 5
        Tcomp1 = value3;
        Tcomp2 = value1;
        Tcomp3 = value2;
    case 4
        Tcomp1 = value3;
        Tcomp2 = value2;
        Tcomp3 = value1;
    case 6
        Tcomp1 = value2;
        Tcomp2 = value3;
        Tcomp3 = value1;
    case 2
        Tcomp1 = value1;
        Tcomp2 = value3;
        Tcomp3 = value2;
end

== matlab function FPC/SVPWM/PWM DutyCaculation ==
  data: CNT input; CH1 output; Tcomp1 input; Tcomp2 input; Tcomp3 input; CH1N output; CH2 output; CH2N output; CH3 output; CH3N output
function [CH1, CH1N, CH2, CH2N, CH3, CH3N] = DutyCaculation(CNT, Tcomp1, Tcomp2, Tcomp3)

% CH1
if CNT < Tcomp1
    CH1 = 0;
    CH1N = 1;
else
    CH1 = 1;
    CH1N = 0;
end

% CH2
if CNT < Tcomp2
    CH2 = 0;
    CH2N = 1;
else
    CH2 = 1;
    CH2N = 0;
end

% CH3
if CNT < Tcomp3
    CH3 = 0;
    CH3N = 1;
else
    CH3 = 1;
    CH3N = 0;
end

== matlab function FPC/SVPWM/PWM SectorJudge ==
  data: A input; N output; B input; C input
function N = SectorJudge(A, B, C)


N = 0;
% if (A > 0)
%     A = 1
% end
% if (A < 0 )
%     A = 0
% end
% if (B > 0)
%     B = 1
% end
% if (B < 0 )
%     B = 0
% end
% if (C > 0)
%     C = 1
% end
% if (C < 0 )
%     C = 0
% end
% N = A + 2*B + 4*C

if (A>0)
    N = N + 1
end
if (B > 0)
    N = N + 2
end
if (C > 0)
    N = N + 4
end

== matlab function FPC/SVPWM/PWM VectorCaculation ==
  data: N input; Ta output; Valpa input; Vbeta input; Udc input; Tpwm input; Tb output
function [Ta, Tb] = SectorCaculation(N, Valpa, Vbeta, Udc, Tpwm)

Ta = double(0);
Tb = double(0);

X = (sqrt(3) * Tpwm) / Udc * Vbeta; % 扇区控制时间 系数1
Y = (sqrt(3) * Tpwm) / Udc * ((sqrt(3) / 2) * Valpa - (1/2) * Vbeta);%  系数2
Z = (sqrt(3) * Tpwm) / Udc * (-(sqrt(3) / 2) * Valpa - (1/2) * Vbeta);%  系数3

if (N == 3)
    Ta = Y;
    Tb = X;
end
if (N == 1) % 偶数扇区 Ta和Tb要交换位置
    Ta = -Y;
    Tb = -Z;
end
if (N == 5)
    Ta = X;
    Tb = Z;
end
if (N == 4)
    Ta = -X;
    Tb = -Y;
end
if (N == 6)
    Ta = Z;
    Tb = Y;
end
if (N == 2)
    Ta = -Z;
    Tb = -X;
end
